simulink model "simulink_rip"  (R2025b)
settings: Solver=VariableStepAuto  StartTime=0.0  StopTime=1000  RelTol=1e-3
values from neighbouring files (symbols this model uses):
  b = 0.004    [rip.m]
  d = 1e-1    (= 0.1)    [rip.m]
  g = 0.04    [rip.m]
  mu = 1e-3    (= 0.001)    [rip.m]
  x0 = [97 3 0]    [rip.m]
settings Model: Creator=robert  LastModifiedBy=robert

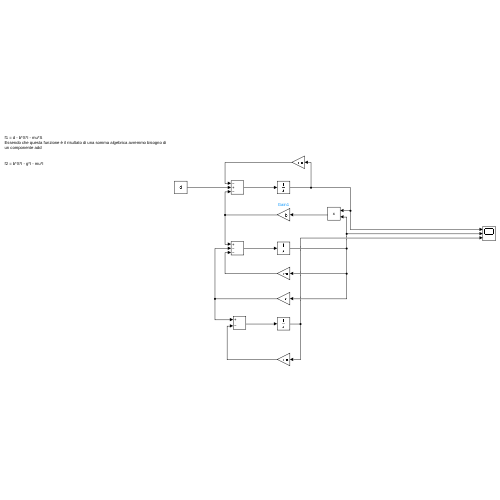
[thumbnail: Simulink's stored preview of the top-level diagram]
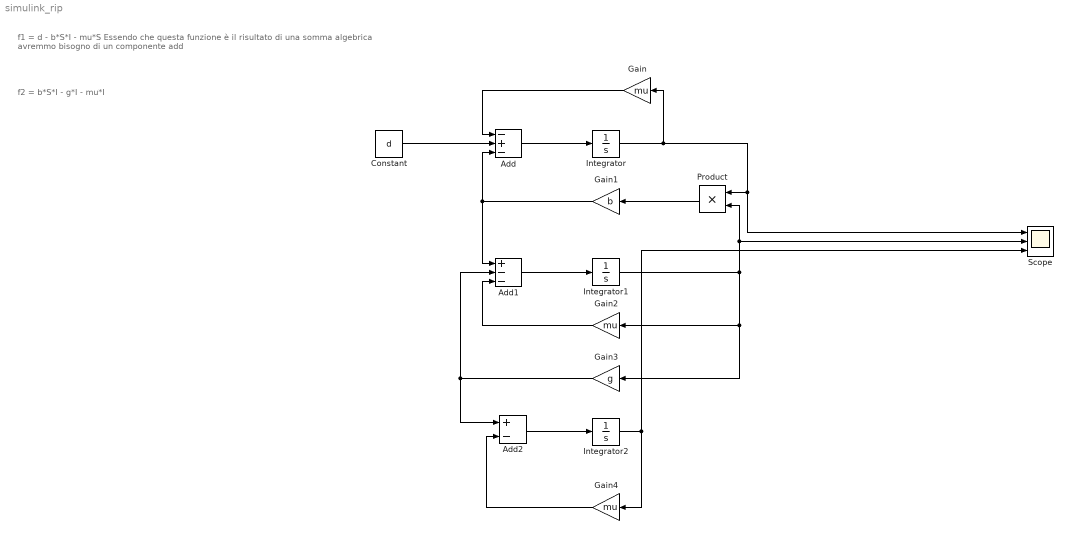
== system simulink_rip ==
  note: f2 = b*S*I - g*I - mu*I
  note: f1 = d - b*S*I - mu*S
      | Essendo che questa funzione è il risultato di una somma algebrica avremmo bisogno di un componente add
  Add : Sum  Inputs=-+-
  Add1 : Sum  Inputs=+--
  Add2 : Sum  Inputs=+-
  Constant : Constant  Value=d
  Gain : Gain  Gain=mu
  Gain1 : Gain  Gain=b
  Gain2 : Gain  Gain=mu
  Gain3 : Gain  Gain=g
  Gain4 : Gain  Gain=mu
  Integrator : Integrator  InitialCondition=x0(1)
  Integrator1 : Integrator  InitialCondition=x0(2)
  Integrator2 : Integrator  InitialCondition=x0(3)
  Product : Product
  Scope : Scope  NumInputPorts=3
      settings: ActiveDisplayYMinimum=-12.124999999999996  ActiveDisplayYMaximum=109.125
  wires:
  Add/1 -> Integrator/1
  Constant/1 -> Add/2
  Integrator/1 -> Scope/1, Product/1, Gain/1
  Gain/1 -> Add/1
  Gain1/1 -> Add1/1, Add/3
  Product/1 -> Gain1/1
  Integrator1/1 -> Scope/2, Product/2, Gain3/1, Gain2/1
  Add1/1 -> Integrator1/1
  Gain2/1 -> Add1/3
  Gain3/1 -> Add2/1, Add1/2
  Add2/1 -> Integrator2/1
  Integrator2/1 -> Scope/3, Gain4/1
  Gain4/1 -> Add2/2
